simulink model "ovr_ut"  (Simulink 8.1)
settings: Solver=FixedStepDiscrete  StartTime=0.0  StopTime=10.0  FixedStep=0.005  RelTol=1e-3
libraries: siltestlib x8, ovr x1
settings Model: Creator=xsellart  LastModifiedBy=AT015555
settings DataIOCC: SignalLoggingSaveFormat=Dataset
settings OptimizationCC: ExpressionDepthLimit=128
settings DebuggingCC: FcnCallInpInsideContextMsg=EnableAllAsError
settings GRTTargetCC: CombineOutputUpdateFcns=on  GRTInterface=off

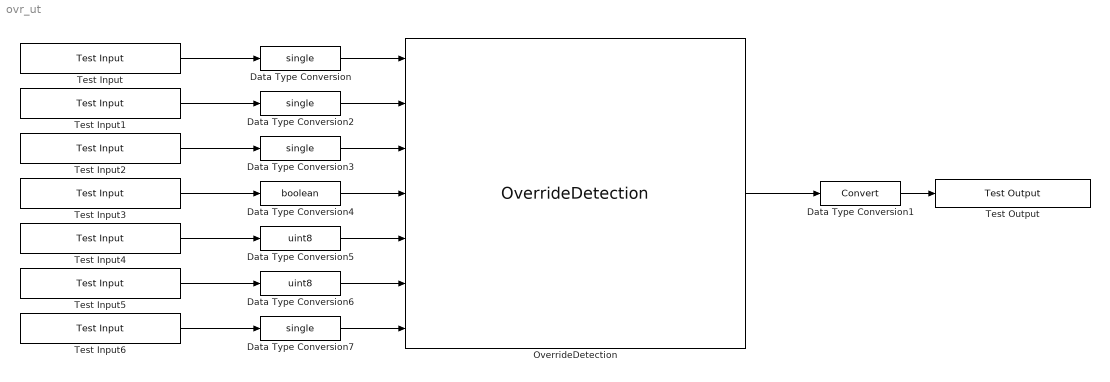
== system ovr_ut ==
  Data Type Conversion{,2..3,7} (4 alike) : DataTypeConversion  OutDataTypeStr=single
  Data Type Conversion1 : DataTypeConversion
  Data Type Conversion4 : DataTypeConversion  OutDataTypeStr=boolean
  Data Type Conversion5 : DataTypeConversion  OutDataTypeStr=uint8
  Data Type Conversion6 : DataTypeConversion  OutDataTypeStr=uint8
  OverrideDetection : ovr/OverrideDetection
  Test Input : siltestlib/Test Input  varname=VDINR_SteerSpeed_degps  sampletime=0.005
  Test Input1 : siltestlib/Test Input  varname=VDINR_HWAccelPedalPosn_pct  sampletime=0.005
  Test Input2 : siltestlib/Test Input  varname=VDINR_SteerAngle_deg  sampletime=0.005
  Test Input3 : siltestlib/Test Input  varname=VDINR_DriverBrakPedalOn_flg  sampletime=0.005
  Test Input4 : siltestlib/Test Input  varname=VFCW_FCWStateHMI_enum  sampletime=0.005
  Test Input5 : siltestlib/Test Input  varname=VAEB_AEBStateHMI_enum  sampletime=0.005
  Test Input6 : siltestlib/Test Input  varname=VDINR_VehSpd_mps  sampletime=0.005
  Test Output : siltestlib/Test Output  varname=VIFO_DriverOverrideReq_flg  sampletime=-1
  wires:
  OverrideDetection/1 -> Data Type Conversion1/1
  Data Type Conversion1/1 -> Test Output/1
  Test Input/1 -> Data Type Conversion/1
  Data Type Conversion/1 -> OverrideDetection/1
  Test Input1/1 -> Data Type Conversion2/1
  Data Type Conversion2/1 -> OverrideDetection/2
  Test Input2/1 -> Data Type Conversion3/1
  Data Type Conversion3/1 -> OverrideDetection/3
  Test Input3/1 -> Data Type Conversion4/1
  Data Type Conversion4/1 -> OverrideDetection/4
  Test Input4/1 -> Data Type Conversion5/1
  Data Type Conversion5/1 -> OverrideDetection/5
  Test Input5/1 -> Data Type Conversion6/1
  Data Type Conversion6/1 -> OverrideDetection/6
  Test Input6/1 -> Data Type Conversion7/1
  Data Type Conversion7/1 -> OverrideDetection/7
